simulink model "Env_cpl_buck_online"  (R2023b)
settings: Solver=VariableStepAuto  StartTime=0.0  StopTime=0.4  RelTol=1e-3
PostLoadFcn:
  | , if any(exist('dsrtsu_mdlpostloadfcn', 'file') == [2, 3, 6]), try dsrtsu_mdlpostloadfcn('Execute', bdroot); catch fprintf('Error in PostLoadFcn (dsrtsu_mdlpostloadfcn) for model "%s":\n %s\n', bdroot, lasterr); end, end,
values from neighbouring files (symbols this model uses):
  C = 0.001    [init.m]
  E = 200    [init.m]
  ESO = 0    [init.m]
  fsw = 2e4    (= 20000)    [init.m]
  initial_power = 200    [init.m]
  Kic = 200    [init.m]
  Kiv = 394    [init.m]
  Kpc = 0.02    [init.m]
  Kpv = 3.3    [init.m]
  L = 0.001    [init.m]
  PI = 1    [init.m]
  Switched_power = 800    [init.m]
  Vref = 100    [init.m]
  w0 = 6000    [init.m]
undefined symbols (not defined in the file or in its folder): h, R, W0
libraries: spsSeriesRLCBranchLib x3, spsControlledCurrentSourceLib x1, spsControlledVoltageSourceLib x1, spsCurrentMeasurementLib x1, spsDiodeLib x1, spsMosfetLib x1, spsPWMGeneratorDCDCLib x1, spsVoltageMeasurementLib x1, sps_lib x1
(part 5 of 5)

== matlab function Env_cpl_buck_online/ESO Fcn ==
  data: yk input; z1_k output; uk input; w0 input; h input; z2_k output; z3_k output
%This function :扩张状态观测器
% Name        : ESO
% Descritions : e = z1 - y
%               z1(k+1) = z1(k) + h*(z2 - β01*e)
%               z2(k+1) = z2(k) + h*(z3 + b*u - β02*e)
%               z3(k+1) = z3(k)  - h*β03*e
% h:采样周期
%β01=3w0，β02=3w0^2，β03=w0^3：控制器参数

function [z1_k,z2_k,z3_k] = ESO(yk,uk,w0,h)
%%  variables definition
persistent  z1_k_1 z2_k_1 z3_k_1
% beta01=30;
% beta02=300;
% beta03=1000;
%J1= 7.061551833333e-6;

%Kt1=0.0384; %kt=1.5*pn*pmsm.fluxPM

%b=Kt1/J1;
% h=0.001;
% alfa1=0.25;
% alfa2=0.5;
% % delta=0.002;
% fal1=1;
% fal2=1;
% b=1;
b=200/(0.001*0.001);
if isempty(z1_k_1)
    z1_k_1=0;
end
if isempty(z2_k_1)
    z2_k_1=0;
end
if isempty(z3_k_1)
    z3_k_1=0;
end
%--------------------------------------------------------------------------
%% 更新变量
e1=z1_k_1-yk;
%限制
z1_k = z1_k_1+h*(z2_k_1-3*w0*e1);
z1_k_1 =double(z1_k); %%迭代更新z1_k_1

%% 更新变量

z2_k=z2_k_1+h*(z3_k_1+b*uk-3*w0*w0*e1);
z2_k_1 = double(z2_k);%%迭代更新z2_k_1


z3_k = z3_k_1-h*w0*w0*w0*e1;
z3_k_1= double(z3_k);%%迭代更新z3_k_1


end
